simulink model "Mass_Flow"  (R2022a)
settings: Solver=FixedStepAuto  StartTime=0.0  StopTime=60.0  RelTol=1e-3  EnableMultiTasking=on
libraries: simulink x3, mbedblockslib x1
settings Model: ExtModeTrigDuration=10  Creator=smith  LastModifiedBy=smith
settings OptimizationCC: EnhancedBackFolding=on  PassReuseOutputArgsAs=Individual arguments  ZeroExternalMemoryAtStartup=off  ZeroInternalMemoryAtStartup=off  MaxStackSize=64  OptimizeBlockOrder=speed  DifferentSizesBufferReuse=on  OptimizationCustomize=off  EfficientTunableParamExpr=on
settings DebuggingCC: ParameterTunabilityLossMsg=error
settings HardwareCC: ProdBitPerPointer=32  ProdBitPerSizeT=32  ProdBitPerPtrDiffT=32  ProdLargestAtomicInteger=Long  ProdLargestAtomicFloat=Double  ProdWordSize=32  ProdLongLongMode=on  ProdHWDeviceType=ARM Compatible->ARM Cortex
settings SFSimCC: MATLABDynamicMemAlloc=off
settings RTWCC: SystemTargetFile=ert.tlc  HardwareBoard=STM32 Nucleo L476RG  TemplateMakefile=ert_default_tmf  Toolchain=GNU Tools for ARM Embedded Processors
settings CodeAppCC: ForceParamTrailComments=on  IgnoreCustomStorageClasses=off  OperatorAnnotations=on  SimulinkDataObjDesc=on  SFDataObjDesc=on  InsertBlockDesc=on
settings ERTTargetCC: SupportContinuousTime=on  ExtModeTransport=3  ExtModeStaticAlloc=on  ExtModeStaticAllocSize=2000  ExtModeMexFile=ext_xcp  ExtModeIntrfLevel=Level2 - Open

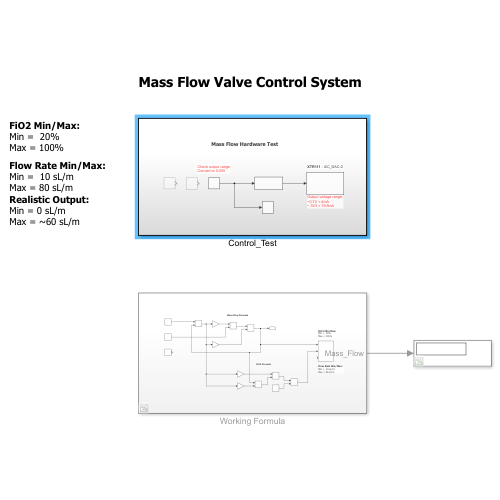
[thumbnail: Simulink's stored preview of the top-level diagram]
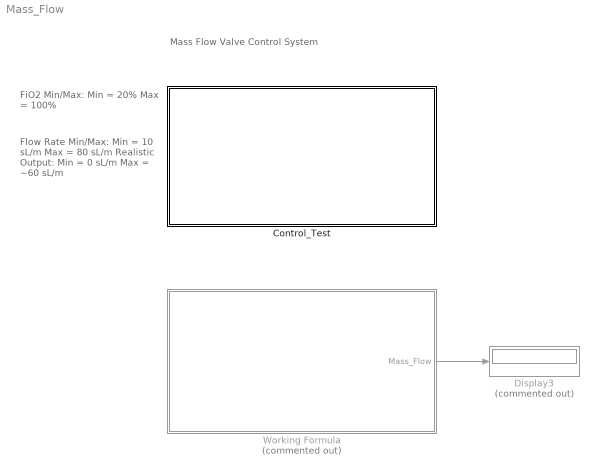
== system Mass_Flow ==
  note: Flow Rate Min/Max:
      | Min = 10 sL/m
      | Max = 80 sL/m
      | Realistic Output:
      | Min = 0 sL/m
      | Max = ~60 sL/m
  note: Mass Flow Valve Control System
  note: FiO2 Min/Max:
      | Min = 20%
      | Max = 100%
  Control_Test : Subsystem
  Display3 : Display  Commented=on
  Working Formula : Subsystem  Commented=on
  wires:
  Working Formula/1(Mass_Flow) -> Display3/1

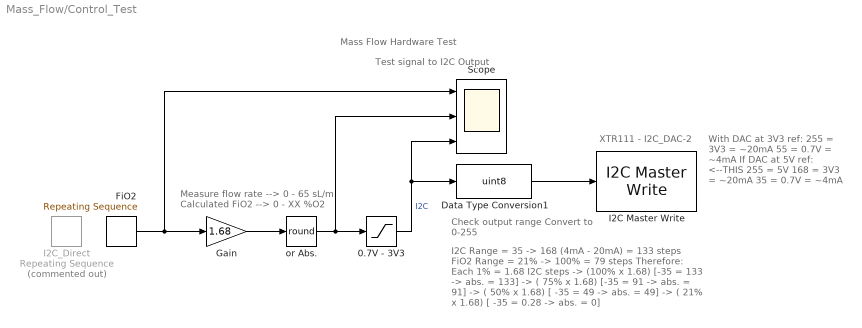
== system Mass_Flow/Control_Test ==
  note: With DAC at 3V3 ref:
      | 255 = 3V3 = ~20mA
      | 55 = 0.7V = ~4mA
      |
      | If DAC at 5V ref: <--THIS
      | 255 = 5V
      | 168 = 3V3 = ~20mA
      | 35 = 0.7V = ~4mA
  note: Check output range
      | Convert to 0-255
  note: Mass Flow Hardware Test
  note: Test signal to I2C Output
  note: XTR111 - I2C_DAC-2
  note: Measure flow rate --> 0 - 65 sL/m
      | Calculated FiO2 --> 0 - XX %O2
  note: I2C Range = 35 -> 168 (4mA - 20mA) = 133 steps
      | FiO2 Range = 21% -> 100% = 79 steps
      | Therefore: Each 1% = 1.68 I2C steps
      |
      | -> (100% x 1.68) [-35 = 133 -> abs. = 133]
      | -> ( 75% x 1.68) [-35 = 91 -> abs. = 91]
      | -> ( 50% x 1.68) [ -35 = 49 -> abs. = 49]
      | -> ( 21% x 1.68) [ -35 = 0.28 -> abs. = 0]
  0.7V - 3V3 : Saturate  UpperLimit=168  LowerLimit=35
  Data Type Conversion1 : DataTypeConversion  OutDataTypeStr=uint8  SaturateOnIntegerOverflow=off  RndMeth=Floor
  FiO2 : simulink/Sources/Repeating Sequence  rep_seq_t=[0 10 10.1 20 20.1 30 30.1 40 40.1 41]  rep_seq_y=[21 21 50 50 100 100 75 75 21 21]
  Gain : Gain  Gain=1.68
  I2C Master Write : mbedblockslib/I2C Master Write  I2CModule=2  Mode=Master  SlaveAddress=uint8(hex2dec('2A'))  SlaveByteOrder=BigEndian  Direction=Transmitter  RegisterAddressMode=on  RegisterAddress=uint8(hex2dec('11'))  SlaveDataType=uint8  DataLength=2  NoAck=off  RepeatedStart=off  OutputStatus=off
      settings: SourceProductBaseCode=MICROBIT,NUCLEO,STMICRODIS
  I2C_Direct : simulink/Sources/Repeating Sequence  Commented=on  rep_seq_t=[0 5 5.1 10 10.1 15 15.1 20 20.1 25]  rep_seq_y=[75 75 120 120 200 200 150 150 75 75]
  Scope : Scope  NumInputPorts=3
  or Abs. : Rounding  Operator=round
  wires:
  Data Type Conversion1/1 -> I2C Master Write/1
  FiO2/1 -> Scope/1, Gain/1
  Gain/1 -> or Abs./1
  0.7V - 3V3/1 -> Scope/3, Data Type Conversion1/1  "I2C"
  or Abs./1 -> Scope/2, 0.7V - 3V3/1

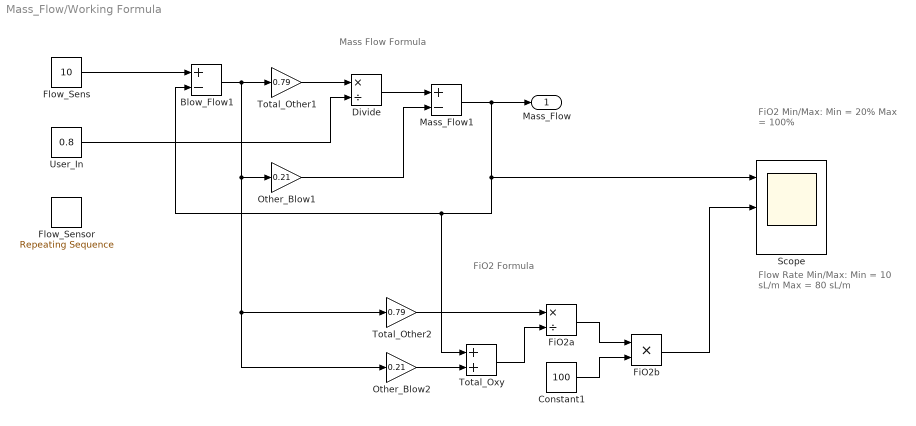
== system Mass_Flow/Working Formula ==
  note: FiO2 Formula
  note: FiO2 Min/Max:
      | Min = 20%
      | Max = 100%
  note: Flow Rate Min/Max:
      | Min = 10 sL/m
      | Max = 80 sL/m
  note: Mass Flow Formula
  Blow_Flow1 : Sum  Inputs=+-
  Constant1 : Constant  Value=100
  Divide : Product  Inputs=*/
  FiO2a : Product  Inputs=*/
  FiO2b : Product
  Flow_Sens : Constant  Value=10
  Flow_Sensor : simulink/Sources/Repeating Sequence  rep_seq_t=[0 1 1.1 2 2.1 3 3.1 4 4.1]  rep_seq_y=[20 20 50 50 35 35 45 45 20]
  Mass_Flow1 : Sum  Inputs=+-
  Other_Blow1 : Gain  Gain=0.21
  Other_Blow2 : Gain  Gain=0.21
  Scope : Scope  NumInputPorts=3
  Total_Other1 : Gain  Gain=0.79
  Total_Other2 : Gain  Gain=0.79
  Total_Oxy : Sum
  User_In : Constant  Value=0.8
  Mass_Flow : Outport
  wires:
  Constant1/1 -> FiO2b/2
  User_In/1 -> Divide/2
  Total_Other1/1 -> Divide/1
  Divide/1 -> Mass_Flow1/1
  Other_Blow1/1 -> Mass_Flow1/2
  Mass_Flow1/1 -> Scope/1, Total_Oxy/1, Blow_Flow1/2, Mass_Flow/1
  FiO2a/1 -> FiO2b/1
  Other_Blow2/1 -> Total_Oxy/2
  Total_Oxy/1 -> FiO2a/2
  Total_Other2/1 -> FiO2a/1
  Flow_Sens/1 -> Blow_Flow1/1
  FiO2b/1 -> Scope/2
  Blow_Flow1/1 -> Other_Blow2/1, Total_Other2/1, Other_Blow1/1, Total_Other1/1
